simulink model "SOB_PMSM_Output_Feedback_20241218"  (R2024b)
settings: Solver=ode1  StartTime=0.0  StopTime=30  FixedStep=1/20000  RelTol=1e-3
values from neighbouring files (symbols this model uses):
  ac1_init = [a1]'    [SOB_PMSM_Fullstate_Feedback_Parameter.m]    (also in SOB_PMSM_Output_Feedback_Parameter.m)
  ac2_init = [a2]'    [SOB_PMSM_Fullstate_Feedback_Parameter.m]    (also in SOB_PMSM_Output_Feedback_Parameter.m)
  ac3_init = [a3]'    [SOB_PMSM_Fullstate_Feedback_Parameter.m]    (also in SOB_PMSM_Output_Feedback_Parameter.m)
  cr1_init = [c1]'    [SOB_PMSM_Fullstate_Feedback_Parameter.m]    (also in SOB_PMSM_Output_Feedback_Parameter.m)
  cr2_init = [c2]'    [SOB_PMSM_Fullstate_Feedback_Parameter.m]    (also in SOB_PMSM_Output_Feedback_Parameter.m)
  cr3_init = [c3]'    [SOB_PMSM_Fullstate_Feedback_Parameter.m]    (also in SOB_PMSM_Output_Feedback_Parameter.m)
  Jm = 4.675e-4    (= 0.0004675)    [SOB_PMSM_Fullstate_Feedback_Parameter.m]    (also in SOB_PMSM_NNSMC_Parameter.m; SOB_PMSM_Output_Feedback_Parameter.m)
  Km = 1.5*Psi*PolePairs    (= 0.102)    [SOB_PMSM_Fullstate_Feedback_Parameter.m]    (also in SOB_PMSM_NNSMC_Parameter.m; SOB_PMSM_Output_Feedback_Parameter.m)
  L = 0.4e-3    (= 0.0004)    [SOB_PMSM_Fullstate_Feedback_Parameter.m]    (also in SOB_PMSM_NNSMC_Parameter.m; SOB_PMSM_Output_Feedback_Parameter.m)
libraries: simulink x1
settings Model: Creator=COLAB  LastModifiedBy=user
settings SolverCC: AlgebraicLoopSolver=TrustRegion
settings RTWCC: GPUComputeCapability=3.5

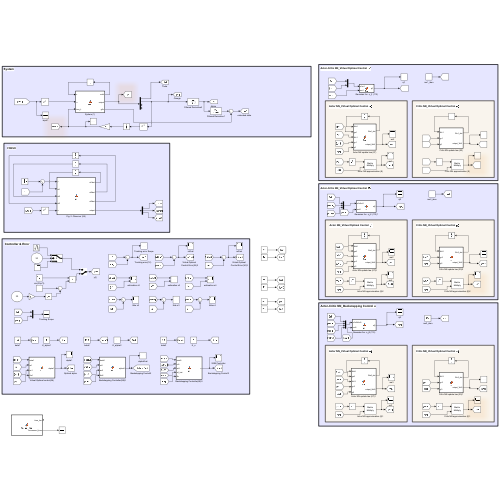
[thumbnail: Simulink's stored preview of the top-level diagram]
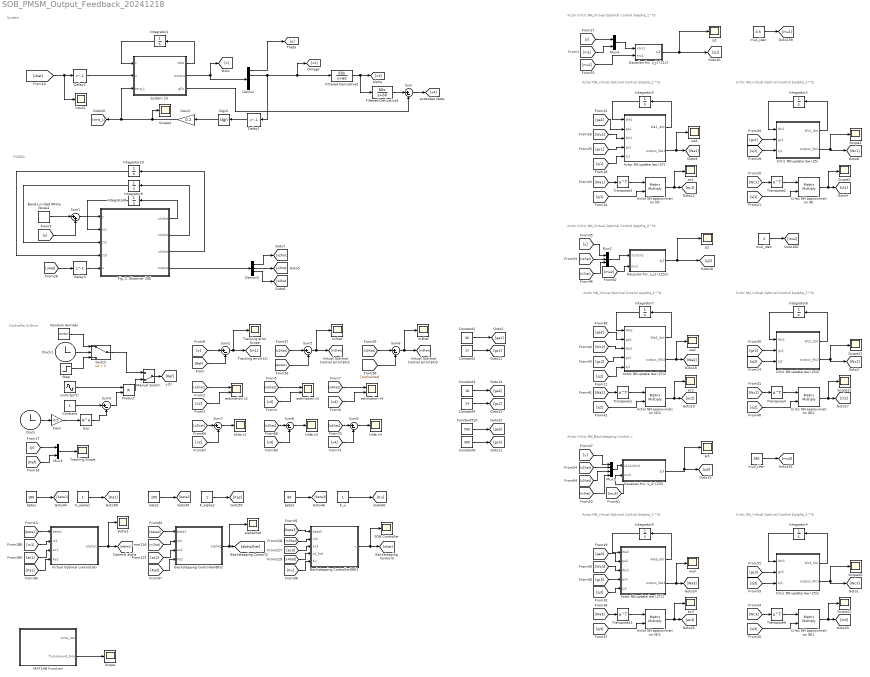
== system SOB_PMSM_Output_Feedback_20241218 ==
  note: System
  note: Controller & Error
  note: Actor-Critic NN_Virtual Optimal Control $\alpha_1^*$
  note: Critic NN_Virtual Optimal Control $\alpha_1^*$
  note: Actor NN_Virtual Optimal Control $\alpha_1^*$
  note: Actor-Critic NN_Backstepping Control u
  note: Critic NN_Virtual Optimal Control $\alpha_1^*$
  note: Actor NN_Virtual Optimal Control $\alpha_1^*$
  note: Actor-Critic NN_Virtual Optimal Control $\alpha_2^*$
  note: Critic NN_Virtual Optimal Control $\alpha_1^*$
  note: Actor NN_Virtual Optimal Control $\alpha_1^*$
  note: FOESO
  Actor NN approximation (8) : Product  Multiplication=Matrix(*)
  Actor NN approximation (8)1 : Product  Multiplication=Matrix(*)
  Actor NN approximation (8)2 : Product  Multiplication=Matrix(*)
  Actor NN update law (27) : MATLAB Function  TreatAsAtomicUnit=on
  Actor NN update law (27)1 : MATLAB Function  TreatAsAtomicUnit=on
  Actor NN update law (27)2 : MATLAB Function  TreatAsAtomicUnit=on
  Backstepping Controller(88)2 : MATLAB Function  TreatAsAtomicUnit=on
  Backstepping Controller(88)3 : MATLAB Function  TreatAsAtomicUnit=on
  Band-Limited White Noise1 : simulink/Sources/Band-Limited White Noise  Cov=1e-7  Ts=1/20000  seed=23341
  Clock : Clock
  Clock1 : Clock
  Constant : Constant
  Constant1 : Constant  Value=30
  Constant2 : Constant  Value=17
  Constant3 : Constant  Value=18
  Constant4 : Constant  Value=14
  Constant510 : Constant  Value=500
  Constant6 : Constant  Value=300
  Critic NN approximation (8) : Product  Multiplication=Matrix(*)
  Critic NN approximation (8)1 : Product  Multiplication=Matrix(*)
  Critic NN approximation (8)2 : Product  Multiplication=Matrix(*)
  Critic NN update law (25) : MATLAB Function  TreatAsAtomicUnit=on
  Critic NN update law (25)1 : MATLAB Function  TreatAsAtomicUnit=on
  Critic NN update law (25)2 : MATLAB Function  TreatAsAtomicUnit=on
  Delay1 : Delay  DelayLength=1
  Delay2 : Delay  DelayLength=1
  Delay3 : Delay  DelayLength=1
  Demux : Demux
  Demux2 : Demux  Outputs=3
  Exp : Math
  Fig. 2. Observer (26) : MATLAB Function  TreatAsAtomicUnit=on
  Filtered Derivative1 : TransferFcn  Numerator=[60 0]  Denominator=[1 60]
  Filtered Derivative2 : TransferFcn  Numerator=[60 0]  Denominator=[1 60]
  Gain : Gain  Gain=-0.5
  Gain2 : Gain  Gain=0.2
  Gaussian fnc. s_j1 (112) : MATLAB Function  TreatAsAtomicUnit=on
  Gaussian fnc. s_j2 (115) : MATLAB Function  TreatAsAtomicUnit=on
  Gaussian fnc. s_j2 (115)1 : MATLAB Function  TreatAsAtomicUnit=on
  Integrator1 : Integrator  InitialCondition=[0 0 0 0]
  Integrator10 : Integrator
  Integrator2 : Integrator  InitialCondition=cr1_init
  Integrator3 : Integrator  InitialCondition=ac1_init
  Integrator4 : Integrator  InitialCondition=cr3_init
  Integrator5 : Integrator  InitialCondition=ac3_init
  Integrator6 : Integrator  InitialCondition=cr2_init
  Integrator7 : Integrator  InitialCondition=ac2_init
  Integrator8 : Integrator
  Integrator9 : Integrator
  K_alpha1 : Constant
  K_alpha2 : Constant
  K_u : Constant
  MATLAB Function : MATLAB Function  TreatAsAtomicUnit=on
  Manual Switch : ManualSwitch  CurrentSetting=0
  Mux1 : Mux
  Mux2 : Mux  Inputs=3
  Mux3 : Mux  Inputs=2
  Mux4 : Mux  Inputs=2
  Product : Product
  Random Number : RandomNumber  Mean=1  Variance=0.05  SampleTime=0.2
  "SOB Controller " : Scope
  Scope{,1..2,4,11..12,20..21} (8 alike) : Scope
  Sign2 : Signum
  Step : Step  SampleTime=0
  Sum{,2..3,5..9} (8 alike) : Sum  Inputs=|+-
  Sum1 : Sum  Inputs=|++
  Switch : Switch  Criteria=u2 > Threshold  Threshold=2  SaturateOnIntegerOverflow=off  InputSameDT=off
  System (1) : MATLAB Function  TreatAsAtomicUnit=on
  Tracking Scope : Scope
  Tracking error Scope : Scope
  Transpose{1..4,9,11} (6 alike) : Math  Operator=transpose  SignedPower=on
  Virtual Optimal control(26) : MATLAB Function  TreatAsAtomicUnit=on
  ac1 : Scope
  ac2 : Scope
  ac3 : Scope
  alpha1 : Scope
  alpha2hat : Scope
  beta1 : Constant  Value=180
  beta2 : Constant  Value=100
  beta3 : Constant  Value=60
  estimation x2 : Scope  NumInputPorts=2
  estimation x3 : Scope  NumInputPorts=2
  estimation x4 : Scope  NumInputPorts=2
  input1 : Scope
  m2hat : Scope
  m3hat : Scope
  mu1_iden : Constant  Value=0.5
  mu2_iden : Constant  Value=3
  mu3_iden : Constant  Value=180
  sin(0.5pi*t) : Sin  Amplitude=2  Frequency=0.5*pi  SampleTime=0
  sj1 : Scope
  sj2 : Scope
  sj3 : Scope
  tilde x2 : Scope
  tilde x3 : Scope
  tilde x4 : Scope
  wa1 : Scope
  wa2 : Scope
  wa3 : Scope
  wires:
  Delay2/1 -> System (1)/2(u)
  Integrator1/1 -> System (1)/1(x)
  [uhat] -> input1/1, Delay2/1
  System (1)/1(xdot) -> Integrator1/1
  Demux/2 -> Delay1/1, Filtered Derivative2/1, [x2]
  Demux/1 -> [y]
  Sign2/1 -> Gain2/1
  Filtered Derivative2/1 -> Filtered Derivative1/1, [x3]
  System (1)/2(output) -> Demux/1, [x]
  Filtered Derivative1/1 -> Sum/1
  System (1)/3(g0u) -> Sum/2
  Sum/1 -> [x4]
  Sum6/1 -> [m3hat], m3hat/1
  [x3hat] -> Sum6/1
  [alpha2hat] -> Sum6/2
  [alpha1] -> Sum5/2
  [x2hat] -> Sum5/1
  Sum5/1 -> m2hat/1, [m2hat]
  sin(0.5pi*t)/1 -> Product/1
  [Ref] -> Sum2/2
  [y] -> Sum2/1
  Sum2/1 -> Tracking error Scope/1, [m1]
  [y] -> Mux3/1
  [Ref] -> Mux3/2
  Mux3/1 -> Tracking Scope/1
  [m3hat] -> Mux1/4
  Gaussian fnc. s_j2 (115)/1(sj3) -> [sj3], sj3/1
  Mux1/1 -> Gaussian fnc. s_j2 (115)/1(x1x2x3m3)
  [x3hat] -> Mux1/3
  [x2hat] -> Mux1/2
  Mux2/1 -> Gaussian fnc. s_j2 (115)1/1(x1x2m2)
  [y] -> Mux2/1
  Gaussian fnc. s_j2 (115)1/1(sj2) -> sj2/1, [sj2]
  [m2hat] -> Mux2/3
  [x2hat] -> Mux2/2
  Critic NN approximation (8)2/1 -> [ct2], Scope12/1
  [sj2] -> Critic NN approximation (8)2/2
  Transpose4/1 -> Critic NN approximation (8)2/1
  [Wc2] -> Transpose4/1
  Critic NN update law (25)2/2(output_Wc2) -> [Wc2], Scope11/1
  [sj2] -> Critic NN update law (25)2/3(sj2)
  Integrator6/1 -> Critic NN update law (25)2/1(Wc2)
  Critic NN update law (25)2/1(Wc2_dot) -> Integrator6/1
  Actor NN update law (27)2/1(Wa2_dot) -> Integrator7/1
  Integrator7/1 -> Actor NN update law (27)2/1(Wa2)
  [sj2] -> Actor NN update law (27)2/5(sj2)
  Actor NN update law (27)2/2(output_Wa2) -> wa2/1, [Wa2]
  [Wa2] -> Transpose1/1
  Transpose1/1 -> Actor NN approximation (8)2/1
  [sj2] -> Actor NN approximation (8)2/2
  Actor NN approximation (8)2/1 -> ac2/1, [ac2]
  [gc2] -> Actor NN update law (27)2/4(gc2)
  [Wc2] -> Actor NN update law (27)2/3(Wc2)
  Critic NN approximation (8)/1 -> [ct1], Scope2/1
  [sj1] -> Critic NN approximation (8)/2
  Transpose2/1 -> Critic NN approximation (8)/1
  [Wc1] -> Transpose2/1
  Critic NN update law (25)/2(output_Wc1) -> [Wc1], Scope1/1
  [sj1] -> Critic NN update law (25)/3(sj1)
  Integrator2/1 -> Critic NN update law (25)/1(Wc1)
  Critic NN update law (25)/1(Wc1_dot) -> Integrator2/1
  Actor NN update law (27)/1(Wa1_dot) -> Integrator3/1
  Integrator3/1 -> Actor NN update law (27)/1(Wa1)
  [sj1] -> Actor NN update law (27)/5(sj1)
  Actor NN update law (27)/2(output_Wa1) -> [Wa1], wa1/1
  [Wa1] -> Transpose3/1
  Transpose3/1 -> Actor NN approximation (8)/1
  [sj1] -> Actor NN approximation (8)/2
  Actor NN approximation (8)/1 -> ac1/1, [ac1]
  [gc1] -> Actor NN update law (27)/4(gc1)
  [Wc1] -> Actor NN update law (27)/3(Wc1)
  [m1] -> Mux4/2
  Mux4/1 -> Gaussian fnc. s_j1 (112)/1(x1m1)
  [y] -> Mux4/1
  Gaussian fnc. s_j1 (112)/1(sj1) -> sj1/1, [sj1]
  [Wc3] -> Actor NN update law (27)1/3(Wc3)
  [gc3] -> Actor NN update law (27)1/4(gc3)
  Actor NN approximation (8)1/1 -> [ac3], ac3/1
  [sj3] -> Actor NN approximation (8)1/2
  Transpose11/1 -> Actor NN approximation (8)1/1
  [Wa3] -> Transpose11/1
  Actor NN update law (27)1/2(output_Wa3) -> wa3/1, [Wa3]
  [sj3] -> Actor NN update law (27)1/5(sj3)
  Integrator5/1 -> Actor NN update law (27)1/1(Wa3)
  Actor NN update law (27)1/1(Wa3_dot) -> Integrator5/1
  Critic NN update law (25)1/1(Wc3_dot) -> Integrator4/1
  Integrator4/1 -> Critic NN update law (25)1/1(Wc3)
  [sj3] -> Critic NN update law (25)1/3(sj3)
  Critic NN update law (25)1/2(output_Wc3) -> [Wc3], Scope20/1
  [Wc3] -> Transpose9/1
  Transpose9/1 -> Critic NN approximation (8)1/1
  [sj3] -> Critic NN approximation (8)1/2
  Critic NN approximation (8)1/1 -> Scope21/1, [ct3]
  [y] -> Mux1/1
  [x4] -> Sum9/2
  Sum9/1 -> tilde x4/1
  [x4hat] -> Sum9/1
  [x3hat] -> Sum8/1
  Sum8/1 -> tilde x3/1
  [x3] -> Sum8/2
  [x2] -> Sum7/2
  Sum7/1 -> tilde x2/1
  [x2hat] -> Sum7/1
  [x4hat] -> estimation x4/1
  [x4] -> estimation x4/2
  [x3] -> estimation x3/2
  [x3hat] -> estimation x3/1
  [x2] -> estimation x2/2
  [x2hat] -> estimation x2/1
  Clock/1 -> Gain/1
  Constant/1 -> Sum3/1
  Exp/1 -> Sum3/2
  Sum3/1 -> Product/2
  Gain/1 -> Exp/1
  [ga1] -> Actor NN update law (27)/2(ga1)
  Constant2/1 -> [gc1]
  [gc1] -> Critic NN update law (25)/2(gc1)
  Constant4/1 -> [gc2]
  Constant3/1 -> [ga2]
  [gc2] -> Critic NN update law (25)2/2(gc2)
  [ga2] -> Actor NN update law (27)2/2(ga2)
  Constant510/1 -> [ga3]
  Constant6/1 -> [gc3]
  [ga3] -> Actor NN update law (27)1/2(ga3)
  [gc3] -> Critic NN update law (25)1/2(gc3)
  [x4hat] -> Backstepping Controller(88)3/4(x4_hat)
  Backstepping Controller(88)2/1(alpha2) -> [alpha2hat], alpha2hat/1
  [Ku] -> Backstepping Controller(88)3/5(Ku)
  [Ka2] -> Backstepping Controller(88)2/4(Ka2)
  [Ka1] -> Virtual Optimal control(26)/4(Ka1)
  K_alpha2/1 -> [Ka2]
  K_alpha1/1 -> [Ka1]
  [beta3] -> Backstepping Controller(88)3/1(beta3)
  [beta2] -> Backstepping Controller(88)2/1(beta2)
  [beta1] -> Virtual Optimal control(26)/1(beta1)
  beta3/1 -> [beta3]
  beta2/1 -> [beta2]
  beta1/1 -> [beta1]
  [m2hat] -> Backstepping Controller(88)2/2(m2)
  [ac2] -> Backstepping Controller(88)2/3(ac2)
  [ac3] -> Backstepping Controller(88)3/3(ac3)
  [m3hat] -> Backstepping Controller(88)3/2(m3)
  Backstepping Controller(88)3/1(u) -> [uhat], "SOB Controller "/1
  [m1] -> Virtual Optimal control(26)/2(m1)
  [ac1] -> Virtual Optimal control(26)/3(ac1)
  Virtual Optimal control(26)/1(alpha1) -> [alpha1], alpha1/1
  Constant1/1 -> [ga1]
  mu1_iden/1 -> [mu1]
  [mu1] -> Gaussian fnc. s_j1 (112)/2(mu1)
  mu2_iden/1 -> [mu2]
  [mu2] -> Gaussian fnc. s_j2 (115)1/2(mu2)
  mu3_iden/1 -> [mu3]
  [mu3] -> Gaussian fnc. s_j2 (115)/2(mu3)
  K_u/1 -> [Ku]
  Gain2/1 -> System (1)/3(torq_L), [torq_L], Scope4/1
  Delay1/1 -> Sign2/1
  Integrator8/1 -> Fig. 2. Observer (26)/2(zt1)
  [uhat] -> Delay3/1
  Demux2/3 -> [x4hat]
  Delay3/1 -> Fig. 2. Observer (26)/5(u)
  Integrator9/1 -> Fig. 2. Observer (26)/3(zt2)
  Fig. 2. Observer (26)/1(zt1dot) -> Integrator8/1
  Integrator10/1 -> Fig. 2. Observer (26)/4(zt3)
  Fig. 2. Observer (26)/3(zt3dot) -> Integrator10/1
  Demux2/2 -> [x3hat]
  Fig. 2. Observer (26)/4(output) -> Demux2/1
  [y] -> Sum1/2
  Fig. 2. Observer (26)/2(zt2dot) -> Integrator9/1
  Band-Limited White Noise1/1 -> Sum1/1
  Demux2/1 -> [x2hat]
  Sum1/1 -> Fig. 2. Observer (26)/1(y)
  MATLAB Function/2(Turnaround_time) -> Scope/1
  Clock1/1 -> Switch/2
  Step/1 -> Switch/3
  Random Number/1 -> Switch/1
  Switch/1 -> Manual Switch/1
  Product/1 -> Manual Switch/2
  Manual Switch/1 -> [Ref]

== matlab function SOB_PMSM_Output_Feedback_20241218/Critic NN update law (25)2 ==
  data: Wc2 input; gc2 input; sj2 input; Wc2_dot output; output_Wc2 output
function [Wc2_dot, output_Wc2] = fcn(Wc2, gc2, sj2)

Wc2_dot = -gc2*sj2*(sj2')*Wc2;

output_Wc2=Wc2;

== matlab function SOB_PMSM_Output_Feedback_20241218/Gaussian fnc. s_j2 (115) ==
  data: x1x2x3m3 input size=4; sj3 output size=16; mean6 parameter; mu3 input
function sj3 = fcn(x1x2x3m3,mean6, mu3)

sjm3=[0 0 0 0 0 0 0 0 0 0 0 0 0 0 0 0];

for i=1:16
    sjm3(i)=gau(i);
end

sj3 = [sjm3]';

function y = gau(x)
    y = exp(-(norm(x1x2x3m3+mean6(x,:)'))^(2)/(mu3^(2)));
end

end

== matlab function SOB_PMSM_Output_Feedback_20241218/Gaussian fnc. s_j1 (112) ==
  data: x1m1 input size=2; sj1 output size=16; mean2 parameter; mu1 input
function sj1 = fcn(x1m1,mean2, mu1)

sjm1=[0 0 0 0 0 0 0 0 0 0 0 0 0 0 0 0];

for i=1:16
    sjm1(i)=gau(i);
end

sj1 = [sjm1]';

function y = gau(x)
    y = exp(-(norm(x1m1+mean2(x,:)'))^(2)/(mu1^(2)));
end

end

== matlab function SOB_PMSM_Output_Feedback_20241218/Critic NN update law (25)1 ==
  data: Wc3 input; gc3 input; sj3 input; Wc3_dot output; output_Wc3 output
function [Wc3_dot, output_Wc3] = fcn(Wc3, gc3, sj3)

Wc3_dot = -gc3*sj3*(sj3')*Wc3;

output_Wc3=Wc3;

== matlab function SOB_PMSM_Output_Feedback_20241218/Gaussian fnc. s_j2 (115)1 ==
  data: x1x2m2 input size=3; sj2 output size=16; mean4 parameter; mu2 input
function sj2  = fcn(x1x2m2,mean4, mu2)

sjm2=[0 0 0 0 0 0 0 0 0 0 0 0 0 0 0 0];

for i=1:16
    sjm2(i)=gau(i);
end

sj2 = [sjm2]';

function y = gau(x)
    y = exp(-(norm(x1x2m2+mean4(x,:)'))^(2)/(mu2^(2)));
end

end

== matlab function SOB_PMSM_Output_Feedback_20241218/Backstepping Controller(88)2 ==
  data: beta2 input; m2 input; alpha2 output; ac2 input; Ka2 input
function alpha2 = fcn(beta2, m2, ac2, Ka2)

alpha2=-beta2*m2-(1/(2*Ka2))*ac2;%-(1/2)*(m2);

== matlab function SOB_PMSM_Output_Feedback_20241218/Backstepping Controller(88)3 ==
  data: beta3 input; m3 input; u output; ac3 input; x4_hat input; Km parameter; Jm parameter; L parameter; Ku input
function u = fcn(beta3, m3, ac3, x4_hat, Km, Jm, L, Ku)

g0=0.1;
u=-(1/(g0*Km/(Jm*L)))*(beta3*m3+(1/(2*Ku))*ac3+x4_hat);

== matlab function SOB_PMSM_Output_Feedback_20241218/Virtual Optimal control(26) ==
  data: beta1 input; m1 input; alpha1 output; ac1 input; Ka1 input
function alpha1 = fcn(beta1, m1, ac1, Ka1)


alpha1=-beta1*m1-(1/(2*Ka1))*ac1;%-(1/2)*(m1);

== matlab function SOB_PMSM_Output_Feedback_20241218/Actor NN update law (27)1 ==
  data: Wa3 input; ga3 input; Wc3 input; gc3 input; sj3 input; Wa3_dot output; output_Wa3 output
function [Wa3_dot, output_Wa3] = fcn(Wa3, ga3, Wc3, gc3, sj3)

Wa3_dot = -sj3*(sj3')*((ga3*(Wa3-Wc3))+gc3*Wc3);

output_Wa3=Wa3;

== matlab function SOB_PMSM_Output_Feedback_20241218/System (1) ==
  data: x input; u input; xdot output; torq_L input; output output; g0u output
function [xdot, output, g0u] = fcn(x, u, torq_L)

Psi       = 0.017;
PolePairs = 4.0;

Km=1.5*Psi*PolePairs;
L=0.4e-3;
J=4.675e-4;
R=0.2;
P=4;
B=2.1e-3;
g0=0.01;

va=-u*sin(P*x(1));
vb=u*cos(P*x(1));
Omega_dot=(1/J)*(-Km*x(3)*sin(P*x(1))+Km*x(4)*cos(P*x(1))-B*x(2)-torq_L);
ia_dot=(1/L)*(va-R*x(3)+Km*x(2)*sin(P*x(1)));
ib_dot=(1/L)*(vb-R*x(4)-Km*x(2)*cos(P*x(1)));

xdot=[x(2) Omega_dot ia_dot ib_dot];

g0u=(g0*Km/(J*L))*u;
output=x;

== matlab function SOB_PMSM_Output_Feedback_20241218/MATLAB Function ==
  data: time_iter output; Turnaround_time output
function [time_iter, Turnaround_time] = toggle_flag()
% time_iter: 0 또는 1로 반복적으로 변하는 출력 변수
% Turnaround_time: 측정된 작업 시간

% Persistent 변수 선언
persistent counter;
persistent stored_Turnaround_time;

% Persistent 변수 초기화
if isempty(counter)
    counter = 0; % 초기 상태 설정
end

if isempty(stored_Turnaround_time)
    stored_Turnaround_time = 0; % 초기 상태 설정
end

% 현재 상태 반환
time_iter = mod(counter, 2); % 0 또는 1을 반환

% Task Turnaround Time 측정
if time_iter == 0
    tic;
    Turnaround_time = stored_Turnaround_time; % 이전 측정값 반환
else
    stored_Turnaround_time = toc;
    Turnaround_time = stored_Turnaround_time; % 현재 측정값 반환
    fprintf('Output Feedback Case Turn around time : %.12f\n', Turnaround_time);
end

% counter 증가
counter = counter + 1;

end

== matlab function SOB_PMSM_Output_Feedback_20241218/Actor NN update law (27)2 ==
  data: Wa2 input; ga2 input; Wc2 input; gc2 input; sj2 input; Wa2_dot output; output_Wa2 output
function [Wa2_dot, output_Wa2] = fcn(Wa2, ga2, Wc2, gc2, sj2)

Wa2_dot = -sj2*(sj2')*((ga2*(Wa2-Wc2))+gc2*Wc2);

output_Wa2=Wa2;

== matlab function SOB_PMSM_Output_Feedback_20241218/Fig. 2. Observer (26) ==
  data: y input; zt1 input; zt1dot output; zt2 input; zt2dot output; zt3 input; zt3dot output; output output; u input; Km parameter; L parameter; Jm parameter
function [zt1dot,zt2dot,zt3dot, output]= fcn(y,zt1,zt2,zt3,u, Km, L, Jm)

g0=0.01; %0.01;

b0=g0*Km/(Jm*L);

M1=1000;
M2=2000;
M3=80000;

l1=1;
l2=1; %4
l3=1;

k1=0.7;
k2=70;

ep=0.01;

%%%%%%%%%%%%%
e1=y-zt1;
zt1dot=(l1*mal(e1))/ep;

v1=zt1dot/M1;

if abs(v1)<1
    min1 = abs(v1);
else
    min1 = 1;
end

sat_v1=sign(v1)*min1;

xhat2=M1*sat_v1;


%%%%%%%%%%%%%%
e2=xhat2-zt2;
zt2dot=(l2*mal(e2))/ep;

v2=zt2dot/M2;

if 1 > abs(v2)
    min2 = abs(v2);
else
    min2 = 1;
end

sat_v2=sign(v2)*min2;

xhat3=M2*sat_v2;

%%%%%%%%%%%%
e3=xhat3-zt3;

zt3dot=((l3*mal(e3))/ep)+b0*u;

v3=((l3*mal(e3))/ep)/M3;

if 1 > abs(v3)
    min3 = abs(v3);
else
    min3 = 1;
end

sat_v3=sign(v3)*min3;

xhat4=M3*sat_v3;

output=[xhat2 xhat3 xhat4];



function y=mal(x)
y=((exp(x)+exp(-x))*x)/(k1*(exp(x)+exp(-x))+k2);
end
end

== matlab function SOB_PMSM_Output_Feedback_20241218/Critic NN update law (25) ==
  data: Wc1 input; gc1 input; sj1 input; Wc1_dot output; output_Wc1 output
function [Wc1_dot, output_Wc1] = fcn(Wc1, gc1, sj1)

Wc1_dot = -gc1*sj1*(sj1')*Wc1;

output_Wc1=Wc1;

== matlab function SOB_PMSM_Output_Feedback_20241218/Actor NN update law (27) ==
  data: Wa1 input; ga1 input; Wc1 input; gc1 input; sj1 input; Wa1_dot output; output_Wa1 output
function [Wa1_dot, output_Wa1] = fcn(Wa1,ga1, Wc1, gc1, sj1)

Wa1_dot = -sj1*(sj1')*((ga1*(Wa1-Wc1))+gc1*Wc1);

output_Wa1=Wa1;
